simulink model "DPSK_2020a"  (R2020a)
settings: Solver=ode45  StartTime=0  StopTime=950  RelTol=1e-3  EnableMultiTasking=on
PreLoadFcn:
  | SNR=7;                           % Signal-to-noise ratio
  | T =  0.1;                         % Symbol period
  | Tc = T/10;                      % Carrier period
  | deltaf = 1e-3/T;               % Frequency error
  | phase = -0.9*pi/2;           % Static phase error
  | Tr=T;                              % cheating ...
  | alpha = 0.18;                   % Rolloff factor
  | warning off all
undefined symbols (not defined in the file or in its folder): alpha, gcbh, rcfiltgaincompat
libraries: commfilt2 x8, dsparch4 x6, commdigbbndpm3 x4, commchan3 x2, commsink2 x2, commrandsrc2 x2
settings Model: Creator=professor  LastModifiedBy=000098944
settings DataIOCC: LimitDataPoints=on  SaveFormat=Array  SignalLoggingSaveFormat=ModelDataLogs  ReturnWorkspaceOutputs=off
settings OptimizationCC: ExpressionDepthLimit=2147483647  InitFltsAndDblsToZero=on  LifeSpan=inf
settings DebuggingCC: AlgebraicLoopMsg=none  SaveWithParameterizedLinksMsg=none  UnderspecifiedInitializationDetection=Classic  MergeDetectMultiDrivingBlocksExec=none  SolverPrmCheckMsg=warning  MultiTaskDSMMsg=warning  MultiTaskCondExecSysMsg=none  FcnCallInpInsideContextMsg=warning  StateNameClashWarn=warning  SFUnexpectedBacktrackingDiag=warning  SFNoUnconditionalDefaultTransitionDiag=warning  SFExecutionAtInitializationDiag=none  ArithmeticOperatorsInVariantConditions=warning
settings HardwareCC: ProdBitPerPointer=32  ProdBitPerSizeT=32  ProdBitPerPtrDiffT=32  ProdLargestAtomicFloat=None  ProdIntDivRoundTo=Undefined  ProdEndianess=Unspecified  ProdWordSize=32  ProdHWDeviceType=32-bit Generic
settings ModelReferenceCC: PropagateSignalLabelsOutOfModel=off
settings SFSimCC: SimUseLocalCustomCode=off  CustomCodeUndefinedFunction=UseInterfaceOnly
settings RTWCC: RTWUseLocalCustomCode=off
settings CodeAppCC: StateflowObjectComments=on
settings GRTTargetCC: TargetFcnLib=ansi_tfl_tmw.mat  TargetLangStandard=C89/C90 (ANSI)  CombineOutputUpdateFcns=off  GRTInterface=on
settings ConfigComp: CovMetricSettings=dw  CovSaveCumulativeToWorkspaceVar=on  CovSaveSingleToWorkspaceVar=on  CovExternalEMLEnable=off  CovSFcnEnable=off

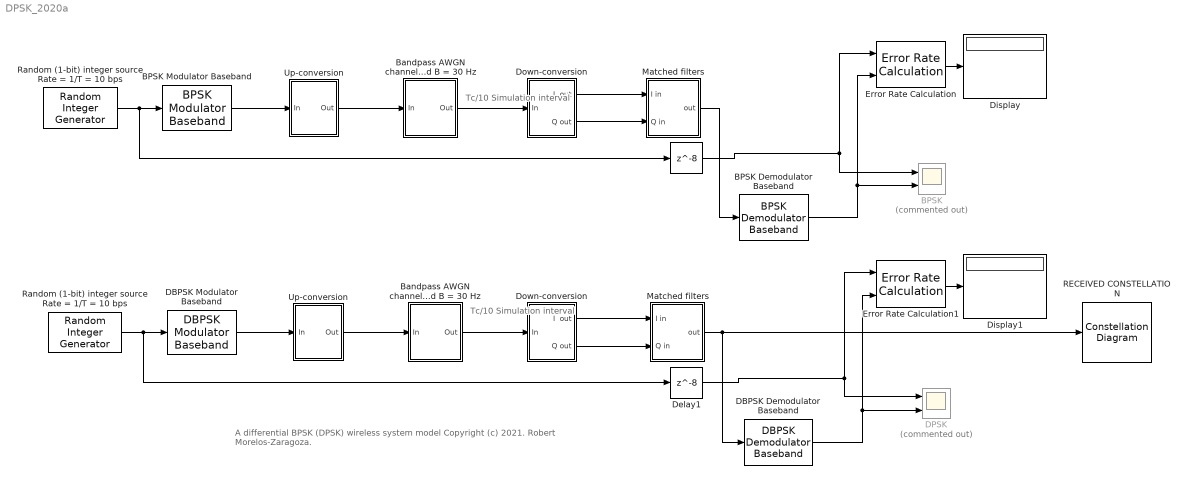
== system DPSK_2020a ==
  note: A differential BPSK (DPSK) wireless system model
      | Copyright (c) 2021. Robert Morelos-Zaragoza.
  note: Tc/10
      |
      | Simulation
      | interval
  note: Tc/10
      |
      | Simulation
      | interval
  " " : Delay  DelayLength=8  InitialCondition=0
  "  Matched filters  " : Subsystem
  " Down-conversion " : Subsystem  TreatAsAtomicUnit=on
  " RECEIVED CONSTELLATION" : ConstellationDiagram  Tag=ScatterPlot
  " Up-conversion " : Subsystem  TreatAsAtomicUnit=on
  BPSK : Scope  Commented=on  NumInputPorts=2
  BPSK Demodulator Baseband : commdigbbndpm3/BPSK Demodulator Baseband  DecType=Hard decision  VarSource=Dialog  Variance=1  Ph=0  outDtype=Inherit via internal rule  derotateFactorWordLen=16  derotateFactorDataTypeStr=Inherit: Same word length as input  derotateFactorLastDataTypeStr=Inherit: Same word length as input
  BPSK Modulator Baseband : commdigbbndpm3/BPSK Modulator Baseband  Ph=0  outDtype=double  outWordLen=16  outUDDataType=sfix(16)  outFracLenMode=Best precision  outFracLen=15  outDataTypeStr=double  outLastDataTypeStr=double
  "Bandpass AWGN channel fc = 100 Hz and B = 30 Hz " : Subsystem  TreatAsAtomicUnit=on
  Bandpass AWGN channel fc = 100 Hz and B = 30 Hz : Subsystem  TreatAsAtomicUnit=on
  DBPSK Demodulator Baseband : commdigbbndpm3/DBPSK Demodulator Baseband  Ph=0  outDtype=Inherit via internal rule
      settings: SourceProductBaseCode=CM
  DBPSK Modulator Baseband : commdigbbndpm3/DBPSK Modulator Baseband  Ph=0  outDtype=double
      settings: SourceProductBaseCode=CM
  DPSK : Scope  Commented=on  NumInputPorts=2
  Delay1 : Delay  DelayLength=8  InitialCondition=0
  Display : Display
  Display1 : Display
  Down-conversion : Subsystem  TreatAsAtomicUnit=on
  Error Rate Calculation : commsink2/Error Rate Calculation  N=0  st_delay=10  cp_mode=Entire frame  subframe=[]  PMode=Port  WsName=ErrorVec  RsMode2=off  stop=off  numErr=100  maxBits=1e6
  Error Rate Calculation1 : commsink2/Error Rate Calculation  N=0  st_delay=10  cp_mode=Entire frame  subframe=[]  PMode=Port  WsName=ErrorVec  RsMode2=off  stop=off  numErr=100  maxBits=1e6
  Matched filters : Subsystem
  "Random (1-bit) integer source Rate = 1/T = 10 bps " : commrandsrc2/Random Integer Generator  mul=2  seed=seed  Ts=T  frameBased=off  sampPerFrame=1  orient=off  outDataType=double
      settings: SourceProductBaseCode=CM
  Random (1-bit) integer source Rate = 1/T = 10 bps : commrandsrc2/Random Integer Generator  mul=2  seed=seed  Ts=T  frameBased=off  sampPerFrame=1  orient=off  outDataType=double
      settings: SourceProductBaseCode=CM
  Up-conversion : Subsystem  TreatAsAtomicUnit=on
  wires:
  Bandpass AWGN channel fc = 100 Hz and B = 30 Hz/1(Out) -> Down-conversion/1(In)
  Down-conversion/1(" I  out ") -> Matched filters/1(I in)
  Down-conversion/2(" Q out ") -> Matched filters/2(Q in)
  Matched filters/1(out) -> BPSK Demodulator Baseband/1
  BPSK Modulator Baseband/1 -> Up-conversion/1(In)
  Random (1-bit) integer source Rate = 1/T = 10 bps/1 -> BPSK Modulator Baseband/1, " "/1
  Up-conversion/1(Out) -> Bandpass AWGN channel fc = 100 Hz and B = 30 Hz/1(In)
  BPSK Demodulator Baseband/1 -> Error Rate Calculation/2, BPSK/2
  " "/1 -> Error Rate Calculation/1, BPSK/1
  DBPSK Modulator Baseband/1 -> " Up-conversion "/1(In)
  Delay1/1 -> Error Rate Calculation1/1, DPSK/1
  "Random (1-bit) integer source Rate = 1/T = 10 bps "/1 -> DBPSK Modulator Baseband/1, Delay1/1
  DBPSK Demodulator Baseband/1 -> Error Rate Calculation1/2, DPSK/2
  " Down-conversion "/2(" Q out ") -> "  Matched filters  "/2(Q in)
  " Up-conversion "/1(Out) -> "Bandpass AWGN channel fc = 100 Hz and B = 30 Hz "/1(In)
  "  Matched filters  "/1(out) -> DBPSK Demodulator Baseband/1, " RECEIVED CONSTELLATION"/1
  " Down-conversion "/1(" I  out ") -> "  Matched filters  "/1(I in)
  "Bandpass AWGN channel fc = 100 Hz and B = 30 Hz "/1(Out) -> " Down-conversion "/1(In)
  Error Rate Calculation/1 -> Display/1
  Error Rate Calculation1/1 -> Display1/1

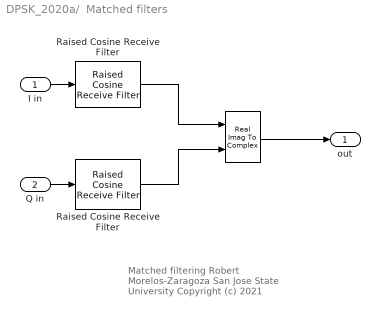
== system DPSK_2020a/  Matched filters   ==
  note: Matched filtering
      |
      | Robert Morelos-Zaragoza
      | San Jose State University
      | Copyright (c) 2021
  I in : Inport
  Q in : Inport  Port=2
  "           " : RealImagToComplex  SampleTime=Tr
  Raised Cosine Receive Filter : commfilt2/Raised Cosine Receive Filter  filtType=Square root  R=alpha  filtSpan=2*(4)  N=4  downFactor=1  downOffset=0  filterGain=(1/2)*rcfiltgaincompat(gcbh)  InputProcessing=Columns as channels (frame based)  RateOptions=Enforce single-rate processing  framing=Mute  checkCoeff=off  variableName=rcRxFilt  currentFiltSpan=2*(4)  D=4  inputOffset=0  sampMode=Mute  saveAsFlag=0  rateMode=Downsampling  checkGain=User-specified  launchFVT=off  roundingMode=Floor  overflowMode=off  coeffDataTypeStr=Inherit: Same word length as input  coeffMin=[]  coeffMax=[]  coeffLastDataTypeStr=Inherit: Same word length as input  accumDataTypeStr=Inherit: Same as product output  accumLastDataTypeStr=Inherit: Same as product output  outputDataTypeStr=Inherit: Same as accumulator  outputMin=[]  outputMax=[]  outputLastDataTypeStr=Inherit: Same as accumulator
  "Raised Cosine Receive Filter " : commfilt2/Raised Cosine Receive Filter  filtType=Square root  R=alpha  filtSpan=2*(4)  N=4  downFactor=1  downOffset=0  filterGain=(1/2)*rcfiltgaincompat(gcbh)  InputProcessing=Columns as channels (frame based)  RateOptions=Enforce single-rate processing  framing=Mute  checkCoeff=off  variableName=rcRxFilt1  currentFiltSpan=2*(4)  D=4  inputOffset=0  sampMode=Mute  saveAsFlag=0  rateMode=Downsampling  checkGain=User-specified  launchFVT=off  roundingMode=Floor  overflowMode=off  coeffDataTypeStr=Inherit: Same word length as input  coeffMin=[]  coeffMax=[]  coeffLastDataTypeStr=Inherit: Same word length as input  accumDataTypeStr=Inherit: Same as product output  accumLastDataTypeStr=Inherit: Same as product output  outputDataTypeStr=Inherit: Same as accumulator  outputMin=[]  outputMax=[]  outputLastDataTypeStr=Inherit: Same as accumulator
  out : Outport
  wires:
  I in/1 -> Raised Cosine Receive Filter/1
  Q in/1 -> "Raised Cosine Receive Filter "/1
  Raised Cosine Receive Filter/1 -> "           "/1
  "Raised Cosine Receive Filter "/1 -> "           "/2
  "           "/1 -> out/1

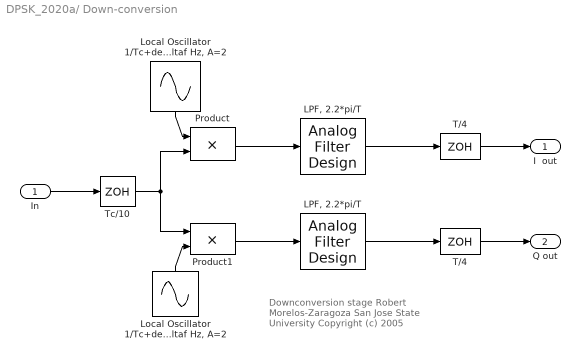
== system DPSK_2020a/ Down-conversion  ==
  note: Downconversion stage
      |
      | Robert Morelos-Zaragoza
      | San Jose State University
      | Copyright (c) 2005
  In : Inport
  " LPF, 2.2*pi/T " : dsparch4/Analog Filter Design  method=Butterworth  filttype=Lowpass  N=7  Wlo=2.2*pi/T  Whi=80  Rp=2  Rs=40
  "LPF, 2.2*pi/T" : dsparch4/Analog Filter Design  method=Butterworth  filttype=Lowpass  N=7  Wlo=2.2*pi/T  Whi=80  Rp=2  Rs=40
  "Local Oscillator 1/Tc+deltaf Hz, A=2 " : Sin  Amplitude=2  Frequency=2*pi/Tc+deltaf  Phase=phase  SampleTime=Tc/10
  "Local Oscillator 1/Tc+deltaf Hz, A=2    " : Sin  Amplitude=2  Frequency=2*pi/Tc+deltaf  Phase=pi/2+phase  SampleTime=Tc/10
  Product : Product  InputSameDT=on  SaturateOnIntegerOverflow=on  OutDataTypeStr=Inherit: Same as first input
  Product1 : Product  InputSameDT=on  SaturateOnIntegerOverflow=on  OutDataTypeStr=Inherit: Same as first input
  T/4 : ZeroOrderHold  SampleTime=T/4
  "T/4 " : ZeroOrderHold  SampleTime=T/4
  Tc/10 : ZeroOrderHold  SampleTime=Tc/10
  " I  out " : Outport
  " Q out " : Outport  Port=2
  wires:
  "Local Oscillator 1/Tc+deltaf Hz, A=2    "/1 -> Product1/2
  "LPF, 2.2*pi/T"/1 -> T/4/1
  "Local Oscillator 1/Tc+deltaf Hz, A=2 "/1 -> Product/1
  Product/1 -> "LPF, 2.2*pi/T"/1
  " LPF, 2.2*pi/T "/1 -> "T/4 "/1
  Product1/1 -> " LPF, 2.2*pi/T "/1
  In/1 -> Tc/10/1
  T/4/1 -> " I  out "/1
  "T/4 "/1 -> " Q out "/1
  Tc/10/1 -> Product/2, Product1/1

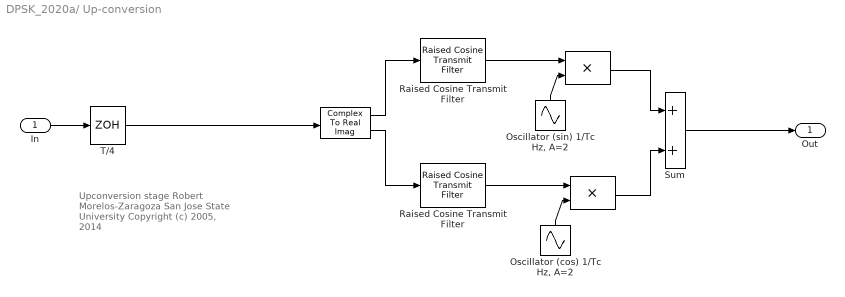
== system DPSK_2020a/ Up-conversion  ==
  note: Upconversion stage
      |
      | Robert Morelos-Zaragoza
      | San Jose State University
      | Copyright (c) 2005, 2014
  In : Inport
  " " : ComplexToRealImag
  "  " : Product  InputSameDT=on  SaturateOnIntegerOverflow=on  OutDataTypeStr=Inherit: Same as first input
  "   " : Product  InputSameDT=on  SaturateOnIntegerOverflow=on  OutDataTypeStr=Inherit: Same as first input
  "Oscillator (cos) 1/Tc Hz, A=2" : Sin  Amplitude=2  Frequency=2*pi/Tc  Phase=pi/2  SampleTime=0
  "Oscillator (sin) 1/Tc Hz, A=2 " : Sin  Amplitude=2  Frequency=2*pi/Tc  SampleTime=0
  Raised Cosine Transmit Filter : commfilt2/Raised Cosine Transmit Filter  filtType=Square root  R=alpha  filtSpan=2*(4)  N=4  filterGain=rcfiltgaincompat(gcbh)  InputProcessing=Columns as channels (frame based)  RateOptions=Allow multirate processing  framing=Mute  checkCoeff=off  variableName=rcTxFilt  checkGain=Normalized  sampMode=Mute  saveAsFlag=0  currentFiltSpan=2*(4)  D=4  launchFVT=off  roundingMode=Floor  overflowMode=off  coeffDataTypeStr=Inherit: Same word length as input  coeffMin=[]  coeffMax=[]  coeffLastDataTypeStr=Inherit: Same word length as input  outputDataTypeStr=Inherit: Same as accumulator  outputMin=[]  outputMax=[]  outputLastDataTypeStr=Inherit: Same as accumulator
  "Raised Cosine Transmit Filter " : commfilt2/Raised Cosine Transmit Filter  filtType=Square root  R=alpha  filtSpan=2*(4)  N=4  filterGain=rcfiltgaincompat(gcbh)  InputProcessing=Columns as channels (frame based)  RateOptions=Allow multirate processing  framing=Mute  checkCoeff=off  variableName=rcTxFilt1  checkGain=Normalized  sampMode=Mute  saveAsFlag=0  currentFiltSpan=2*(4)  D=4  launchFVT=off  roundingMode=Floor  overflowMode=off  coeffDataTypeStr=Inherit: Same word length as input  coeffMin=[]  coeffMax=[]  coeffLastDataTypeStr=Inherit: Same word length as input  outputDataTypeStr=Inherit: Same as accumulator  outputMin=[]  outputMax=[]  outputLastDataTypeStr=Inherit: Same as accumulator
  Sum : Sum  InputSameDT=on  SaturateOnIntegerOverflow=on  OutDataTypeStr=Inherit: Same as first input
  T/4 : ZeroOrderHold  SampleTime=T/4
  Out : Outport
  wires:
  In/1 -> T/4/1
  Raised Cosine Transmit Filter/1 -> "  "/1
  "Raised Cosine Transmit Filter "/1 -> "   "/1
  "Oscillator (sin) 1/Tc Hz, A=2 "/1 -> "  "/2
  "Oscillator (cos) 1/Tc Hz, A=2"/1 -> "   "/2
  "  "/1 -> Sum/1
  "   "/1 -> Sum/2
  Sum/1 -> Out/1
  " "/1 -> Raised Cosine Transmit Filter/1
  " "/2 -> "Raised Cosine Transmit Filter "/1
  T/4/1 -> " "/1

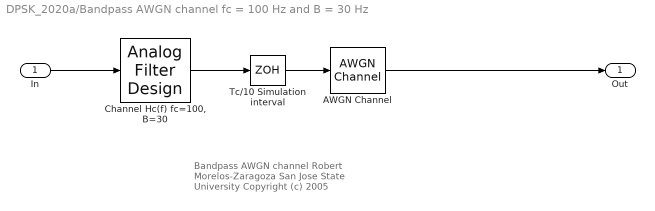
== system DPSK_2020a/Bandpass AWGN channel fc = 100 Hz and B = 30 Hz  ==
  note: Bandpass AWGN channel
      |
      | Robert Morelos-Zaragoza
      | San Jose State University
      | Copyright (c) 2005
  In : Inport
  AWGN Channel : commchan3/AWGN Channel  InputProcessing=Columns as channels (frame based)  seed=seed  noiseMode="Signal to noise ratio  (Es/No)"  EbNodB=SNR  EsNodB=SNR  SNRdB=SNR  bitsPerSym=2  Ps=1.3  Tsym=T/4  variance=1
  "Channel Hc(f) fc=100, B=30" : dsparch4/Analog Filter Design  method=Chebyshev I  filttype=Bandpass  N=20  Wlo=2*pi*85  Whi=2*pi*115  Rp=0.5  Rs=30
  Tc/10 Simulation interval : ZeroOrderHold  SampleTime=Tc/10
  Out : Outport
  wires:
  "Channel Hc(f) fc=100, B=30"/1 -> Tc/10 Simulation interval/1
  AWGN Channel/1 -> Out/1
  In/1 -> "Channel Hc(f) fc=100, B=30"/1
  Tc/10 Simulation interval/1 -> AWGN Channel/1

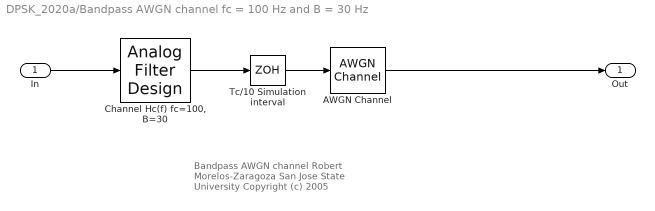
== system DPSK_2020a/Bandpass AWGN channel fc = 100 Hz and B = 30 Hz ==
  note: Bandpass AWGN channel
      |
      | Robert Morelos-Zaragoza
      | San Jose State University
      | Copyright (c) 2005
  In : Inport
  AWGN Channel : commchan3/AWGN Channel  InputProcessing=Columns as channels (frame based)  seed=seed  noiseMode="Signal to noise ratio  (Es/No)"  EbNodB=SNR  EsNodB=SNR  SNRdB=SNR  bitsPerSym=2  Ps=1.3  Tsym=T/4  variance=1
  "Channel Hc(f) fc=100, B=30" : dsparch4/Analog Filter Design  method=Chebyshev I  filttype=Bandpass  N=20  Wlo=2*pi*85  Whi=2*pi*115  Rp=0.5  Rs=30
  Tc/10 Simulation interval : ZeroOrderHold  SampleTime=Tc/10
  Out : Outport
  wires:
  "Channel Hc(f) fc=100, B=30"/1 -> Tc/10 Simulation interval/1
  AWGN Channel/1 -> Out/1
  In/1 -> "Channel Hc(f) fc=100, B=30"/1
  Tc/10 Simulation interval/1 -> AWGN Channel/1

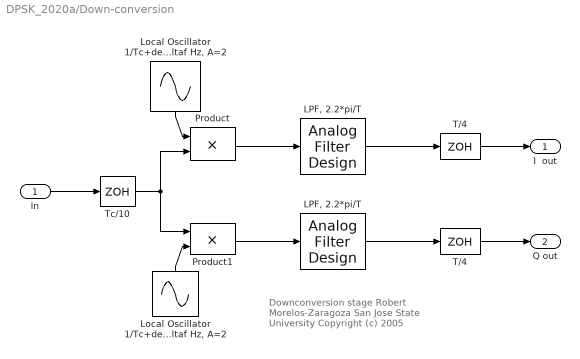
== system DPSK_2020a/Down-conversion ==
  note: Downconversion stage
      |
      | Robert Morelos-Zaragoza
      | San Jose State University
      | Copyright (c) 2005
  In : Inport
  " LPF, 2.2*pi/T " : dsparch4/Analog Filter Design  method=Butterworth  filttype=Lowpass  N=7  Wlo=2.2*pi/T  Whi=80  Rp=2  Rs=40
  "LPF, 2.2*pi/T" : dsparch4/Analog Filter Design  method=Butterworth  filttype=Lowpass  N=7  Wlo=2.2*pi/T  Whi=80  Rp=2  Rs=40
  "Local Oscillator 1/Tc+deltaf Hz, A=2 " : Sin  Amplitude=2  Frequency=2*pi/Tc+deltaf  Phase=phase  SampleTime=Tc/10
  "Local Oscillator 1/Tc+deltaf Hz, A=2    " : Sin  Amplitude=2  Frequency=2*pi/Tc+deltaf  Phase=pi/2+phase  SampleTime=Tc/10
  Product : Product  InputSameDT=on  SaturateOnIntegerOverflow=on  OutDataTypeStr=Inherit: Same as first input
  Product1 : Product  InputSameDT=on  SaturateOnIntegerOverflow=on  OutDataTypeStr=Inherit: Same as first input
  T/4 : ZeroOrderHold  SampleTime=T/4
  "T/4 " : ZeroOrderHold  SampleTime=T/4
  Tc/10 : ZeroOrderHold  SampleTime=Tc/10
  " I  out " : Outport
  " Q out " : Outport  Port=2
  wires:
  "Local Oscillator 1/Tc+deltaf Hz, A=2    "/1 -> Product1/2
  "LPF, 2.2*pi/T"/1 -> T/4/1
  "Local Oscillator 1/Tc+deltaf Hz, A=2 "/1 -> Product/1
  Product/1 -> "LPF, 2.2*pi/T"/1
  " LPF, 2.2*pi/T "/1 -> "T/4 "/1
  Product1/1 -> " LPF, 2.2*pi/T "/1
  In/1 -> Tc/10/1
  T/4/1 -> " I  out "/1
  "T/4 "/1 -> " Q out "/1
  Tc/10/1 -> Product/2, Product1/1

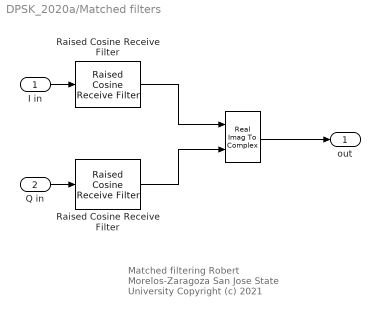
== system DPSK_2020a/Matched filters ==
  note: Matched filtering
      |
      | Robert Morelos-Zaragoza
      | San Jose State University
      | Copyright (c) 2021
  I in : Inport
  Q in : Inport  Port=2
  "           " : RealImagToComplex  SampleTime=Tr
  Raised Cosine Receive Filter : commfilt2/Raised Cosine Receive Filter  filtType=Square root  R=alpha  filtSpan=2*(4)  N=4  downFactor=1  downOffset=0  filterGain=(1/2)*rcfiltgaincompat(gcbh)  InputProcessing=Columns as channels (frame based)  RateOptions=Enforce single-rate processing  framing=Mute  checkCoeff=off  variableName=rcRxFilt  currentFiltSpan=2*(4)  D=4  inputOffset=0  sampMode=Mute  saveAsFlag=0  rateMode=Downsampling  checkGain=User-specified  launchFVT=off  roundingMode=Floor  overflowMode=off  coeffDataTypeStr=Inherit: Same word length as input  coeffMin=[]  coeffMax=[]  coeffLastDataTypeStr=Inherit: Same word length as input  accumDataTypeStr=Inherit: Same as product output  accumLastDataTypeStr=Inherit: Same as product output  outputDataTypeStr=Inherit: Same as accumulator  outputMin=[]  outputMax=[]  outputLastDataTypeStr=Inherit: Same as accumulator
  "Raised Cosine Receive Filter " : commfilt2/Raised Cosine Receive Filter  filtType=Square root  R=alpha  filtSpan=2*(4)  N=4  downFactor=1  downOffset=0  filterGain=(1/2)*rcfiltgaincompat(gcbh)  InputProcessing=Columns as channels (frame based)  RateOptions=Enforce single-rate processing  framing=Mute  checkCoeff=off  variableName=rcRxFilt1  currentFiltSpan=2*(4)  D=4  inputOffset=0  sampMode=Mute  saveAsFlag=0  rateMode=Downsampling  checkGain=User-specified  launchFVT=off  roundingMode=Floor  overflowMode=off  coeffDataTypeStr=Inherit: Same word length as input  coeffMin=[]  coeffMax=[]  coeffLastDataTypeStr=Inherit: Same word length as input  accumDataTypeStr=Inherit: Same as product output  accumLastDataTypeStr=Inherit: Same as product output  outputDataTypeStr=Inherit: Same as accumulator  outputMin=[]  outputMax=[]  outputLastDataTypeStr=Inherit: Same as accumulator
  out : Outport
  wires:
  I in/1 -> Raised Cosine Receive Filter/1
  Q in/1 -> "Raised Cosine Receive Filter "/1
  Raised Cosine Receive Filter/1 -> "           "/1
  "Raised Cosine Receive Filter "/1 -> "           "/2
  "           "/1 -> out/1

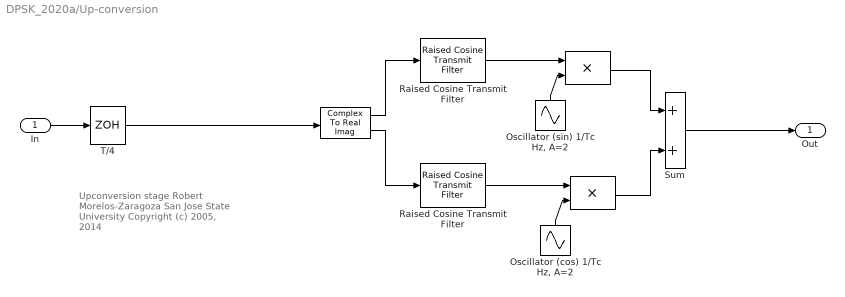
== system DPSK_2020a/Up-conversion ==
  note: Upconversion stage
      |
      | Robert Morelos-Zaragoza
      | San Jose State University
      | Copyright (c) 2005, 2014
  In : Inport
  " " : ComplexToRealImag
  "  " : Product  InputSameDT=on  SaturateOnIntegerOverflow=on  OutDataTypeStr=Inherit: Same as first input
  "   " : Product  InputSameDT=on  SaturateOnIntegerOverflow=on  OutDataTypeStr=Inherit: Same as first input
  "Oscillator (cos) 1/Tc Hz, A=2" : Sin  Amplitude=2  Frequency=2*pi/Tc  Phase=pi/2  SampleTime=0
  "Oscillator (sin) 1/Tc Hz, A=2 " : Sin  Amplitude=2  Frequency=2*pi/Tc  SampleTime=0
  Raised Cosine Transmit Filter : commfilt2/Raised Cosine Transmit Filter  filtType=Square root  R=alpha  filtSpan=2*(4)  N=4  filterGain=rcfiltgaincompat(gcbh)  InputProcessing=Columns as channels (frame based)  RateOptions=Allow multirate processing  framing=Mute  checkCoeff=off  variableName=rcTxFilt  checkGain=Normalized  sampMode=Mute  saveAsFlag=0  currentFiltSpan=2*(4)  D=4  launchFVT=off  roundingMode=Floor  overflowMode=off  coeffDataTypeStr=Inherit: Same word length as input  coeffMin=[]  coeffMax=[]  coeffLastDataTypeStr=Inherit: Same word length as input  outputDataTypeStr=Inherit: Same as accumulator  outputMin=[]  outputMax=[]  outputLastDataTypeStr=Inherit: Same as accumulator
  "Raised Cosine Transmit Filter " : commfilt2/Raised Cosine Transmit Filter  filtType=Square root  R=alpha  filtSpan=2*(4)  N=4  filterGain=rcfiltgaincompat(gcbh)  InputProcessing=Columns as channels (frame based)  RateOptions=Allow multirate processing  framing=Mute  checkCoeff=off  variableName=rcTxFilt1  checkGain=Normalized  sampMode=Mute  saveAsFlag=0  currentFiltSpan=2*(4)  D=4  launchFVT=off  roundingMode=Floor  overflowMode=off  coeffDataTypeStr=Inherit: Same word length as input  coeffMin=[]  coeffMax=[]  coeffLastDataTypeStr=Inherit: Same word length as input  outputDataTypeStr=Inherit: Same as accumulator  outputMin=[]  outputMax=[]  outputLastDataTypeStr=Inherit: Same as accumulator
  Sum : Sum  InputSameDT=on  SaturateOnIntegerOverflow=on  OutDataTypeStr=Inherit: Same as first input
  T/4 : ZeroOrderHold  SampleTime=T/4
  Out : Outport
  wires:
  In/1 -> T/4/1
  Raised Cosine Transmit Filter/1 -> "  "/1
  "Raised Cosine Transmit Filter "/1 -> "   "/1
  "Oscillator (sin) 1/Tc Hz, A=2 "/1 -> "  "/2
  "Oscillator (cos) 1/Tc Hz, A=2"/1 -> "   "/2
  "  "/1 -> Sum/1
  "   "/1 -> Sum/2
  Sum/1 -> Out/1
  " "/1 -> Raised Cosine Transmit Filter/1
  " "/2 -> "Raised Cosine Transmit Filter "/1
  T/4/1 -> " "/1
